simulink model "sim_punto_5"  (R2021b)
settings: Solver=VariableStepAuto  StartTime=0.0  StopTime=30  RelTol=1e-3
values from neighbouring files (symbols this model uses):
  A = [0 1 0 0 0 0 0 0 0 0 0 0 ... (first row only)    [punto5.m]
  B = [0; 0; 0; 0; 0; 0; 0; 0; 0; 0; 0; 1]    [punto5.m]
  C = [1 0 0 0 0 0 0 0 0 0 0 0]    [punto5.m]
  C_states = eye(12)    [punto5.m]
  D_states = [0 0 0 0 0 0 0 0 0 0 0 0]'    [punto5.m]
  N3 = 100    [punto5.m]
  Q = [1+q 0 0 0 0 0 0 0 0 0 0 0 ... (first row only)    [punto5.m]
  R = r    (= 1e-05)    [punto5.m]
  S = [0 0 0 0 0 0 0 0 0 0 0 0 ... (first row only)    [punto5.m]
  Ts = 0.1    [punto5.m]
  U_max = 15    [punto5.m]
  U_min = -15    [punto5.m]
  Ubar = inv(g)*Ybar    [punto5.m]
  umax = 15    [punto5.m]
  umin = -15    [punto5.m]
  x0 = [9 0 9 0 9 0 9 0 9 0 9 0]'    [punto5.m]
  Xbar = -inv(A) * B * Ubar    [punto5.m]
  xmax = [repmat(xmax,N,1)]    [mympc_constraints.m]    (also in punto5.m = [10 inf 10 inf 10 inf 10 inf 10 inf 10 inf]')
  xmin = [repmat(xmin,N,1)]    [mympc_constraints.m]    (also in punto5.m = [-10 -inf -10 -inf -10 -inf -10 -inf -10 -inf -10 -inf]')
undefined symbols (not defined in the file or in its folder): mympc, mympc_constraints
settings Model: Creator=danie  LastModifiedBy=danie

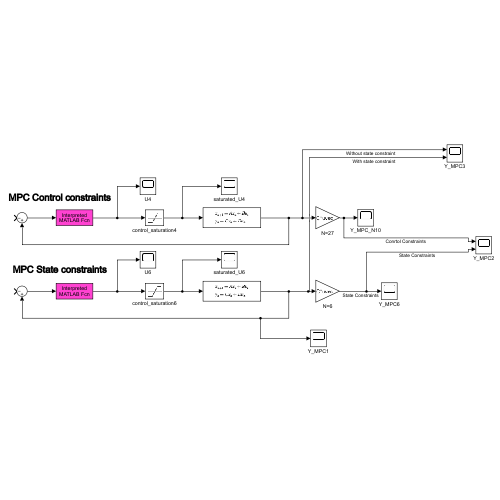
[thumbnail: Simulink's stored preview of the top-level diagram]
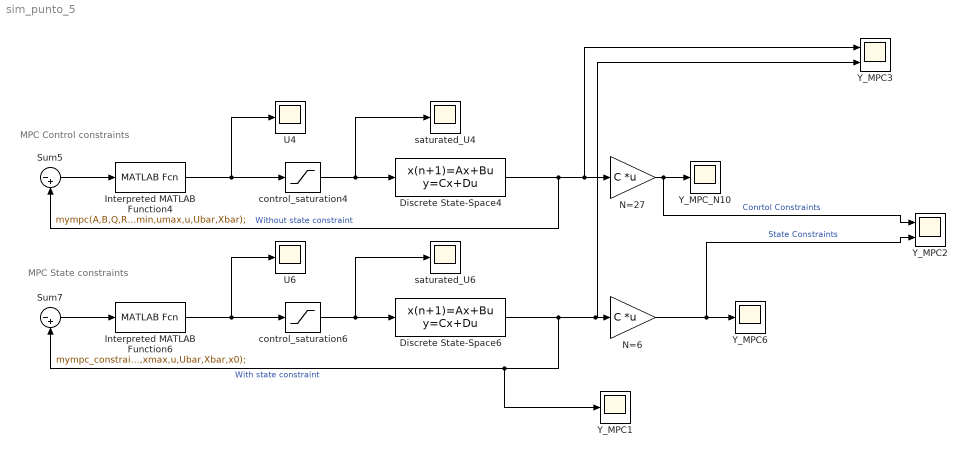
== system sim_punto_5 ==
  note: MPC State constraints
  note: MPC Control constraints
  Discrete State-Space4 : DiscreteStateSpace  A=A  B=B  C=C_states  D=D_states  InitialCondition=x0  SampleTime=Ts
  Discrete State-Space6 : DiscreteStateSpace  A=A  B=B  C=C_states  D=D_states  InitialCondition=x0  SampleTime=Ts
  Interpreted MATLAB Function4 : MATLABFcn  MATLABFcn=mympc(A,B,Q,R,S,N3,umin,umax,u,Ubar,Xbar);  OutputDimensions=1
  Interpreted MATLAB Function6 : MATLABFcn  MATLABFcn=mympc_constraints(A,B,Q,R,S,N3,umin,umax,xmin,xmax,u,Ubar,Xbar,x0);  OutputDimensions=1
  N=27 : Gain  Gain=C  Multiplication=Matrix(K*u) (u vector)
  N=6 : Gain  Gain=C  Multiplication=Matrix(K*u) (u vector)
  Sum5 : Sum  Inputs=|-+
  Sum7 : Sum  Inputs=|-+
  U4 : Scope
  U6 : Scope
  Y_MPC1 : Scope
  Y_MPC2 : Scope  NumInputPorts=2
  Y_MPC3 : Scope  NumInputPorts=2
  Y_MPC6 : Scope
  Y_MPC_N10 : Scope
  control_saturation4 : Saturate  UpperLimit=U_max  LowerLimit=U_min
  control_saturation6 : Saturate  UpperLimit=inf  LowerLimit=-inf
  saturated_U4 : Scope
  saturated_U6 : Scope
  wires:
  Discrete State-Space6/1 -> Y_MPC1/1, Sum7/2, Y_MPC3/2, N=6/1  "With state constraint"
  control_saturation6/1 -> saturated_U6/1, Discrete State-Space6/1
  Sum7/1 -> Interpreted MATLAB Function6/1
  Interpreted MATLAB Function6/1 -> control_saturation6/1, U6/1
  N=6/1 -> Y_MPC2/2, Y_MPC6/1  "State Constraints"
  N=27/1 -> Y_MPC2/1, Y_MPC_N10/1  "Conrtol Constraints"
  Interpreted MATLAB Function4/1 -> control_saturation4/1, U4/1
  Discrete State-Space4/1 -> Sum5/2, Y_MPC3/1, N=27/1  "Without state constraint"
  control_saturation4/1 -> saturated_U4/1, Discrete State-Space4/1
  Sum5/1 -> Interpreted MATLAB Function4/1
